simulink library "speedgoatlib_mscp"  (R2024b)
settings: Solver=VariableStepAuto  StartTime=0.0  StopTime=10.0  RelTol=1e-3
libraries: slrealtimeethercatlib x517, simulink x316, hdlsllib x168, $bdroot x11, slrealtimeutilitieslib x1
(part 1 of 5)
settings Model: Creator=lars.brockmann  LastModifiedBy=speedgoat\jenkins
settings ConfigComp: CovBoundaryAbsTol=1.0e-5

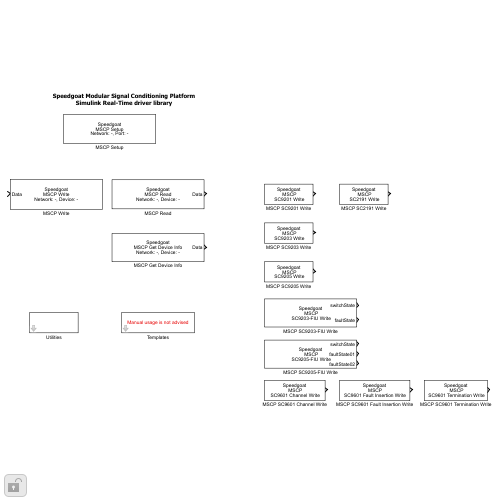
[thumbnail: Simulink's stored preview of the top-level diagram]
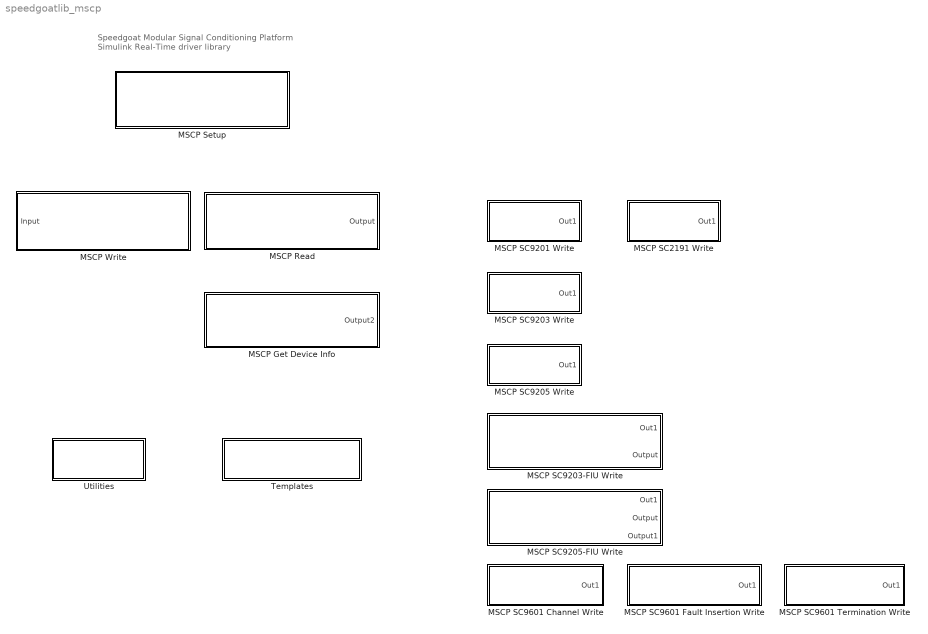
== system speedgoatlib_mscp ==
  note: Speedgoat Modular Signal Conditioning Platform
      | Simulink Real-Time driver library
  MSCP Get Device Info : Subsystem  mask(mscp_getDeviceInfo){}
      settings: OpenFcn=sg_mscp.mask.openFcn('MSCP Get Device Info');
      mask Help: eval('sg.utils.help.show(''io_main/refentry_mscp_get_device_info'');')
      mask Display: disp('Speedgoat\nMSCP Get Device Info\nNetwork: -, Device: -');port_label('output',1,'Data');
  MSCP Read : Subsystem  mask(mscp_read){}
      settings: OpenFcn=sg_mscp.mask.openFcn('MSCP Read');
      mask Help: eval('sg.utils.help.show(''io_main/refentry_mscp_read'');')
      mask Display: disp('Speedgoat\nMSCP Read\nNetwork: -, Device: -');port_label('output',1,'Data');
  MSCP SC2191 Write : Subsystem  mask(mscp_sc2191_write){}
      settings: OpenFcn=sg_mscp.mask.openFcn('MSCP SC2191 Write')
      mask Help: eval('sg.utils.help.show(''io_main/refentry_mscp_sc2191'');')
      mask Display: disp('Speedgoat\n MSCP\n SC2191 Write')
  MSCP SC9201 Write : Subsystem  mask(mscp_sc9201_write){switchState=0}
      settings: OpenFcn=sg_mscp.mask.openFcn(['MSCP SC9201 Write (',gcb,')'])
      mask Help: eval('sg.utils.help.show(''io_main/refentry_mscp_sc9201'');')
      mask Display: disp('Speedgoat\n MSCP\n SC9201 Write')
  MSCP SC9203 Write : Subsystem  mask(mscp_sc9203_write){switchState=0}
      settings: OpenFcn=sg_mscp.mask.openFcn(['MSCP SC9203 Write (',gcb,')'])
      mask Help: eval('sg.utils.help.show(''io_main/refentry_mscp_sc9203'');')
      mask Display: disp('Speedgoat\n MSCP\n SC9203 Write')
  MSCP SC9203-FIU Write : Subsystem  mask(mscp_sc9203_fiu_write){switchState=0, faultState=0}
      settings: OpenFcn=sg_mscp.mask.openFcn(['MSCP SC9203-FIU Write (',gcb,')'])
      mask Help: eval('sg.utils.help.show(''io_main/refentry_mscp_sc9203_fiu'');')
      mask Display:
      | port_label('output', 1, 'switchState');
      | port_label('output', 2, 'faultState');
      | disp('Speedgoat\n MSCP\n SC9203-FIU Write')
  MSCP SC9205 Write : Subsystem  mask(mscp_sc9205_write){switchState=0}
      settings: OpenFcn=sg_mscp.mask.openFcn(['MSCP SC9205 Write (',gcb,')'])
      mask Help: eval('sg.utils.help.show(''io_main/refentry_mscp_sc9205'');')
      mask Display: disp('Speedgoat\n MSCP\n SC9205 Write')
  MSCP SC9205-FIU Write : Subsystem  mask(mscp_sc9205_fiu_write){switchState=0, faultState01=0, faultState02=0}
      settings: OpenFcn=sg_mscp.mask.openFcn(['MSCP SC9205-FIU Write (',gcb,')'])
      mask Help: eval('sg.utils.help.show(''io_main/refentry_mscp_sc9205_fiu'');')
      mask Display:
      | port_label('output', 1, 'switchState');
      | port_label('output', 2, 'faultState01');
      | port_label('output', 3, 'faultState02');
      | disp('Speedgoat\n MSCP\n SC9205-FIU Write')
  MSCP SC9601 Channel Write : Subsystem  mask(mscp_sc9601_channel_write){switchState=0}
      settings: OpenFcn=sg_mscp.mask.openFcn;
      mask Help: eval('sg.utils.help.show(''io_main/refentry_ref_mscp'');')
      mask Display: disp('Speedgoat\n MSCP\n SC9601 Channel Write')
  MSCP SC9601 Fault Insertion Write : Subsystem  mask(mscp_sc9601_fault_insertion_write){switchState=0}
      settings: OpenFcn=sg_mscp.mask.openFcn;
      mask Help: eval('sg.utils.help.show(''io_main/refentry_ref_mscp'');')
      mask Display: disp('Speedgoat\n MSCP\n SC9601 Fault Insertion Write')
  MSCP SC9601 Termination Write : Subsystem  mask(mscp_sc9601_termination_write){switchState=0}
      settings: OpenFcn=sg_mscp.mask.openFcn;
      mask Help: eval('sg.utils.help.show(''io_main/refentry_ref_mscp'');')
      mask Display: disp('Speedgoat\n MSCP\n SC9601 Termination Write')
  MSCP Setup : Subsystem  mask(mscp_setup){}
      settings: OpenFcn=sg_mscp.mask.openFcn('MSCP Setup');
      mask Help: eval('sg.utils.help.show(''io_main/refentry_mscp_setup'');')
      mask Display: disp('Speedgoat\nMSCP Setup\nNetwork: -, Port: -');
  MSCP Write : Subsystem  mask(mscp_write){}
      settings: OpenFcn=sg_mscp.mask.openFcn('MSCP Write');
      mask Help: eval('sg.utils.help.show(''io_main/refentry_mscp_write'');')
      mask Display: disp('Speedgoat\nMSCP Write\nNetwork: -, Device: -');port_label('input',1,'Data');
  Templates : Subsystem
      mask Display:
      | color('red');
      | disp('Manual usage is not advised');
  Utilities : Subsystem

== system speedgoatlib_mscp/MSCP Get Device Info ==
  Bus Creator : BusCreator  Inputs=12
  Subsystem Device : Subsystem  Commented=on
  Subsystem Slot 01 : Subsystem  Commented=on
  Subsystem Slot 02 : Subsystem  Commented=on
  Subsystem Slot 03 : Subsystem  Commented=on
  Subsystem Slot 04 : Subsystem  Commented=on
  Subsystem Slot 05 : Subsystem  Commented=on
  Subsystem Slot 06 : Subsystem  Commented=on
  Subsystem Slot 07 : Subsystem  Commented=on
  Subsystem Slot 08 : Subsystem  Commented=on
  Subsystem Slot 09 : Subsystem  Commented=on
  Subsystem Slot 10 : Subsystem  Commented=on
  Subsystem Slot 11 : Subsystem  Commented=on
  Output2 : Outport
  wires:
  Subsystem Slot 01/1(Out1) -> Bus Creator/2  "Slot_01"
  Subsystem Slot 02/1(Out1) -> Bus Creator/3  "Slot_02"
  Subsystem Slot 03/1(Out1) -> Bus Creator/4  "Slot_03"
  Subsystem Slot 04/1(Out1) -> Bus Creator/5  "Slot_04"
  Subsystem Slot 05/1(Out1) -> Bus Creator/6  "Slot_05"
  Subsystem Slot 06/1(Out1) -> Bus Creator/7  "Slot_06"
  Subsystem Slot 07/1(Out1) -> Bus Creator/8  "Slot_07"
  Subsystem Slot 08/1(Out1) -> Bus Creator/9  "Slot_08"
  Subsystem Slot 09/1(Out1) -> Bus Creator/10  "Slot_09"
  Subsystem Slot 10/1(Out1) -> Bus Creator/11  "Slot_10"
  Subsystem Slot 11/1(Out1) -> Bus Creator/12  "Slot_11"
  Bus Creator/1 -> Output2/1  "Data"
  Subsystem Device/1(Out1) -> Bus Creator/1  "Device"

== system speedgoatlib_mscp/MSCP Read ==
  Output : Outport

== system speedgoatlib_mscp/MSCP SC2191 Write ==
  Configuration : Constant  Value=0  OutDataTypeStr=Bus: MscpBus_SC2191_Write
  Out1 : Outport
  wires:
  Configuration/1 -> Out1/1

== system speedgoatlib_mscp/MSCP SC9201 Write ==
  Constant : Constant  Value=switchState  OutDataTypeStr=uint8
  Out1 : Outport
  wires:
  Constant/1 -> Out1/1

== system speedgoatlib_mscp/MSCP SC9203 Write ==
  Constant : Constant  Value=switchState  OutDataTypeStr=uint8
  Out1 : Outport
  wires:
  Constant/1 -> Out1/1

== system speedgoatlib_mscp/MSCP SC9203-FIU Write ==
  Constant : Constant  Value=switchState  OutDataTypeStr=uint8
  Constant1 : Constant  Value=faultState  OutDataTypeStr=uint8
  Out1 : Outport
  Output : Outport  Port=2
  wires:
  Constant/1 -> Out1/1
  Constant1/1 -> Output/1

== system speedgoatlib_mscp/MSCP SC9205 Write ==
  Constant : Constant  Value=switchState  OutDataTypeStr=uint8
  Out1 : Outport
  wires:
  Constant/1 -> Out1/1

== system speedgoatlib_mscp/MSCP SC9205-FIU Write ==
  Constant : Constant  Value=switchState  OutDataTypeStr=uint8
  Constant1 : Constant  Value=faultState01  OutDataTypeStr=uint8
  Constant2 : Constant  Value=faultState02  OutDataTypeStr=uint8
  Out1 : Outport
  Output : Outport  Port=2
  Output1 : Outport  Port=3
  wires:
  Constant1/1 -> Output/1
  Constant/1 -> Out1/1
  Constant2/1 -> Output1/1

== system speedgoatlib_mscp/MSCP SC9601 Channel Write ==
  Constant : Constant  Value=switchState  OutDataTypeStr=uint8
  Out1 : Outport
  wires:
  Constant/1 -> Out1/1

== system speedgoatlib_mscp/MSCP SC9601 Fault Insertion Write ==
  Constant : Constant  Value=switchState  OutDataTypeStr=uint8
  Out1 : Outport
  wires:
  Constant/1 -> Out1/1

== system speedgoatlib_mscp/MSCP SC9601 Termination Write ==
  Constant : Constant  Value=switchState  OutDataTypeStr=uint8
  Out1 : Outport
  wires:
  Constant/1 -> Out1/1

== system speedgoatlib_mscp/MSCP Setup ==
  Constant : Constant
  Terminator : Terminator
  wires:
  Constant/1 -> Terminator/1

== system speedgoatlib_mscp/MSCP Write ==
  Input : Inport
  Terminator : Terminator
  wires:
  Input/1 -> Terminator/1

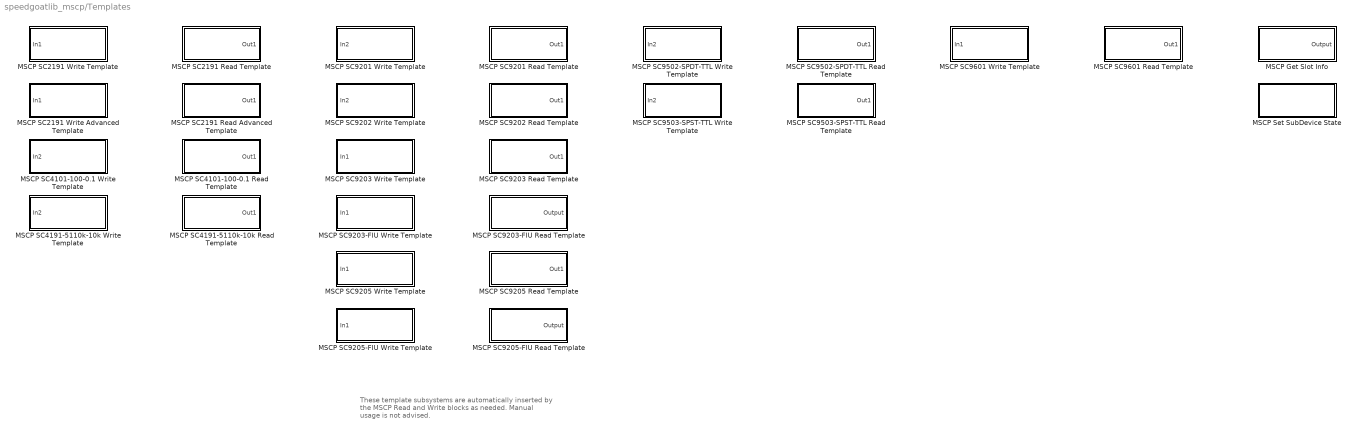
== system speedgoatlib_mscp/Templates ==
  note: These template subsystems are automatically inserted
      | by the MSCP Read and Write blocks as needed.
      | Manual usage is not advised.
  MSCP Get Slot Info : Subsystem
  MSCP SC2191 Read Advanced Template : Subsystem
  MSCP SC2191 Read Template : Subsystem
  MSCP SC2191 Write Advanced Template : Subsystem
  MSCP SC2191 Write Template : Subsystem
  MSCP SC4101-100-0.1 Read Template : Subsystem
  MSCP SC4101-100-0.1 Write Template : Subsystem
  MSCP SC4191-5110k-10k Read Template : Subsystem
  MSCP SC4191-5110k-10k Write Template : Subsystem
  MSCP SC9201 Read Template : Subsystem
  MSCP SC9201 Write Template : Subsystem
  MSCP SC9202 Read Template : Subsystem
  MSCP SC9202 Write Template : Subsystem
  MSCP SC9203 Read Template : Subsystem
  MSCP SC9203 Write Template : Subsystem
  MSCP SC9203-FIU Read Template : Subsystem
  MSCP SC9203-FIU Write Template : Subsystem
  MSCP SC9205 Read Template : Subsystem
  MSCP SC9205 Write Template : Subsystem
  MSCP SC9205-FIU Read Template : Subsystem
  MSCP SC9205-FIU Write Template : Subsystem
  MSCP SC9502-SPDT-TTL Read Template : Subsystem
  MSCP SC9502-SPDT-TTL Write Template : Subsystem
  MSCP SC9503-SPST-TTL Read Template : Subsystem
  MSCP SC9503-SPST-TTL Write Template : Subsystem
  MSCP SC9601 Read Template : Subsystem
  MSCP SC9601 Write Template : Subsystem
  MSCP Set SubDevice State : Subsystem

== system speedgoatlib_mscp/Utilities ==
  MSCP Parse Emergency : S-Function  FunctionName=sg_mscp_parse_ecat_emergency  SFunctionDeploymentMode=off  EnableBusSupport=off
  MSCP Parse Notifications : S-Function  FunctionName=sg_mscp_parse_ecat_notifications  SFunctionDeploymentMode=off  EnableBusSupport=off

== system speedgoatlib_mscp/MSCP Get Device Info/Subsystem Device ==
  ASCII to String : ASCIIToString
  ASCII to String1 : ASCIIToString
  Bus Creator : BusCreator  Inputs=2
  Cast : DataTypeConversion  OutDataTypeStr=int32  SaturateOnIntegerOverflow=off  RndMeth=Floor
  Compare To Constant : simulink/Logic and Bit Operations/Compare To Constant  relop=>=  const=2  OutDataTypeStr=boolean
  EtherCAT Async SDO Upload 0x1008 : slrealtimeethercatlib/EtherCAT Async SDO Upload  index=0  subIndex=0  sig_type=uint8  sig_dim=16  device_id=0  sample_time=1  subdevice_addr=0  selected_subdevice=Term 1 (EK1100)  timeout=500  subdevice_found=0  complete=0
  EtherCAT Async SDO Upload 0x100A : slrealtimeethercatlib/EtherCAT Async SDO Upload  index=0  subIndex=0  sig_type=uint8  sig_dim=16  device_id=0  sample_time=1  subdevice_addr=0  selected_subdevice=Term 1 (EK1100)  timeout=500  subdevice_found=0  complete=0
  Get SubDevice State : slrealtimeethercatlib/Get SubDevice State  device_id=0  sample_time=1  subdevice_addr=0  selected_subdevice=Term 1 (EK1100)  timeout=500  subdevice_found=0
  Terminator{2..5} (4 alike) : Terminator
  Out1 : Outport
  wires:
  Bus Creator/1 -> Out1/1
  EtherCAT Async SDO Upload 0x100A/3 -> Terminator2/1
  EtherCAT Async SDO Upload 0x100A/2 -> Terminator3/1
  EtherCAT Async SDO Upload 0x1008/3 -> Terminator4/1
  EtherCAT Async SDO Upload 0x1008/2 -> Terminator5/1
  Get SubDevice State/1 -> Compare To Constant/1
  Compare To Constant/1 -> Cast/1
  Cast/1 -> EtherCAT Async SDO Upload 0x1008/1, EtherCAT Async SDO Upload 0x100A/1
  ASCII to String/1 -> Bus Creator/2  "Software Version"
  EtherCAT Async SDO Upload 0x100A/1 -> ASCII to String/1
  ASCII to String1/1 -> Bus Creator/1  "Manufacturer Device Name"
  EtherCAT Async SDO Upload 0x1008/1 -> ASCII to String1/1

== system speedgoatlib_mscp/MSCP Get Device Info/Subsystem Slot 01 ==
  MSCP Get Slot Info : $bdroot/Templates/MSCP Get Slot Info  SystemSampleTime=-1  VariantActivationTime=update diagram  EmptyChoice=off  PassThrough=off  PassThroughVariantControl=(default)  EmptyChoiceVariantControl=(default)  AllowFlexibleInterface=on  Latency=0  AutoFrameSizeCalculation=off
  Out1 : Outport
  wires:
  MSCP Get Slot Info/1 -> Out1/1

== system speedgoatlib_mscp/MSCP Get Device Info/Subsystem Slot 02 ==
  MSCP Get Slot Info : $bdroot/Templates/MSCP Get Slot Info  SystemSampleTime=-1  VariantActivationTime=update diagram  EmptyChoice=off  PassThrough=off  PassThroughVariantControl=(default)  EmptyChoiceVariantControl=(default)  AllowFlexibleInterface=on  Latency=0  AutoFrameSizeCalculation=off
  Out1 : Outport
  wires:
  MSCP Get Slot Info/1 -> Out1/1

== system speedgoatlib_mscp/MSCP Get Device Info/Subsystem Slot 03 ==
  MSCP Get Slot Info : $bdroot/Templates/MSCP Get Slot Info  SystemSampleTime=-1  VariantActivationTime=update diagram  EmptyChoice=off  PassThrough=off  PassThroughVariantControl=(default)  EmptyChoiceVariantControl=(default)  AllowFlexibleInterface=on  Latency=0  AutoFrameSizeCalculation=off
  Out1 : Outport
  wires:
  MSCP Get Slot Info/1 -> Out1/1

== system speedgoatlib_mscp/MSCP Get Device Info/Subsystem Slot 04 ==
  MSCP Get Slot Info : $bdroot/Templates/MSCP Get Slot Info  SystemSampleTime=-1  VariantActivationTime=update diagram  EmptyChoice=off  PassThrough=off  PassThroughVariantControl=(default)  EmptyChoiceVariantControl=(default)  AllowFlexibleInterface=on  Latency=0  AutoFrameSizeCalculation=off
  Out1 : Outport
  wires:
  MSCP Get Slot Info/1 -> Out1/1

== system speedgoatlib_mscp/MSCP Get Device Info/Subsystem Slot 05 ==
  MSCP Get Slot Info : $bdroot/Templates/MSCP Get Slot Info  SystemSampleTime=-1  VariantActivationTime=update diagram  EmptyChoice=off  PassThrough=off  PassThroughVariantControl=(default)  EmptyChoiceVariantControl=(default)  AllowFlexibleInterface=on  Latency=0  AutoFrameSizeCalculation=off
  Out1 : Outport
  wires:
  MSCP Get Slot Info/1 -> Out1/1

== system speedgoatlib_mscp/MSCP Get Device Info/Subsystem Slot 06 ==
  MSCP Get Slot Info : $bdroot/Templates/MSCP Get Slot Info  SystemSampleTime=-1  VariantActivationTime=update diagram  EmptyChoice=off  PassThrough=off  PassThroughVariantControl=(default)  EmptyChoiceVariantControl=(default)  AllowFlexibleInterface=on  Latency=0  AutoFrameSizeCalculation=off
  Out1 : Outport
  wires:
  MSCP Get Slot Info/1 -> Out1/1

== system speedgoatlib_mscp/MSCP Get Device Info/Subsystem Slot 07 ==
  MSCP Get Slot Info : $bdroot/Templates/MSCP Get Slot Info  SystemSampleTime=-1  VariantActivationTime=update diagram  EmptyChoice=off  PassThrough=off  PassThroughVariantControl=(default)  EmptyChoiceVariantControl=(default)  AllowFlexibleInterface=on  Latency=0  AutoFrameSizeCalculation=off
  Out1 : Outport
  wires:
  MSCP Get Slot Info/1 -> Out1/1

== system speedgoatlib_mscp/MSCP Get Device Info/Subsystem Slot 08 ==
  MSCP Get Slot Info : $bdroot/Templates/MSCP Get Slot Info  SystemSampleTime=-1  VariantActivationTime=update diagram  EmptyChoice=off  PassThrough=off  PassThroughVariantControl=(default)  EmptyChoiceVariantControl=(default)  AllowFlexibleInterface=on  Latency=0  AutoFrameSizeCalculation=off
  Out1 : Outport
  wires:
  MSCP Get Slot Info/1 -> Out1/1

== system speedgoatlib_mscp/MSCP Get Device Info/Subsystem Slot 09 ==
  MSCP Get Slot Info : $bdroot/Templates/MSCP Get Slot Info  SystemSampleTime=-1  VariantActivationTime=update diagram  EmptyChoice=off  PassThrough=off  PassThroughVariantControl=(default)  EmptyChoiceVariantControl=(default)  AllowFlexibleInterface=on  Latency=0  AutoFrameSizeCalculation=off
  Out1 : Outport
  wires:
  MSCP Get Slot Info/1 -> Out1/1

== system speedgoatlib_mscp/MSCP Get Device Info/Subsystem Slot 10 ==
  MSCP Get Slot Info : $bdroot/Templates/MSCP Get Slot Info  SystemSampleTime=-1  VariantActivationTime=update diagram  EmptyChoice=off  PassThrough=off  PassThroughVariantControl=(default)  EmptyChoiceVariantControl=(default)  AllowFlexibleInterface=on  Latency=0  AutoFrameSizeCalculation=off
  Out1 : Outport
  wires:
  MSCP Get Slot Info/1 -> Out1/1

== system speedgoatlib_mscp/MSCP Get Device Info/Subsystem Slot 11 ==
  MSCP Get Slot Info : $bdroot/Templates/MSCP Get Slot Info  SystemSampleTime=-1  VariantActivationTime=update diagram  EmptyChoice=off  PassThrough=off  PassThroughVariantControl=(default)  EmptyChoiceVariantControl=(default)  AllowFlexibleInterface=on  Latency=0  AutoFrameSizeCalculation=off
  Out1 : Outport
  wires:
  MSCP Get Slot Info/1 -> Out1/1

== system speedgoatlib_mscp/Templates/MSCP Get Slot Info ==
  ASCII to String{,1..3} (4 alike) : ASCIIToString
  Bus Creator : BusCreator  Inputs=9
  Byte Unpacking : slrealtimeutilitieslib/Byte Unpacking  MaskUnpackedDataTypes={'uint16', 'boolean', 'uint8', 'uint8', 'uint8', 'uint32','uint8', 'int64', 'uint8', 'uint16'}  MaskUnpackedDataSizes={[1], [1], [1], [32], [64], [1], [16], [1], [32],[1]}  MaskAlignment=1
  Cast : DataTypeConversion  OutDataTypeStr=int32  SaturateOnIntegerOverflow=off  RndMeth=Floor
  Compare To Constant : simulink/Logic and Bit Operations/Compare To Constant  relop=>=  const=2  OutDataTypeStr=boolean
  EtherCAT Async SDO Upload : slrealtimeethercatlib/EtherCAT Async SDO Upload  index=0  subIndex=0  sig_type=uint8  sig_dim=162  device_id=0  sample_time=1  subdevice_addr=0  selected_subdevice=Term 1 (EK1100)  timeout=500  subdevice_found=0  complete=0
  Get SubDevice State : slrealtimeethercatlib/Get SubDevice State  device_id=0  sample_time=1  subdevice_addr=0  selected_subdevice=Term 1 (EK1100)  timeout=500  subdevice_found=0
  Terminator : Terminator
  Terminator1 : Terminator
  Terminator2 : Terminator
  To String : ToString
  Output : Outport
  wires:
  Cast/1 -> EtherCAT Async SDO Upload/1
  Get SubDevice State/1 -> Compare To Constant/1
  Compare To Constant/1 -> Cast/1
  EtherCAT Async SDO Upload/2 -> Terminator1/1
  Byte Unpacking/3 -> Bus Creator/2  "Header Layout Version"
  Byte Unpacking/1 -> Terminator/1  "number of subobjects"
  EtherCAT Async SDO Upload/3 -> Terminator2/1
  Byte Unpacking/6 -> Bus Creator/5  "Module Identificaiton Number"
  Byte Unpacking/2 -> Bus Creator/1  "Header Control Byte"
  EtherCAT Async SDO Upload/1 -> Byte Unpacking/1
  ASCII to String/1 -> Bus Creator/4  "Notes"
  Byte Unpacking/5 -> ASCII to String/1
  Bus Creator/1 -> Output/1
  Byte Unpacking/7 -> ASCII to String1/1
  ASCII to String1/1 -> Bus Creator/6  "Hardware Version"
  Byte Unpacking/4 -> ASCII to String2/1
  ASCII to String2/1 -> Bus Creator/3  "Product Name"
  Byte Unpacking/8 -> To String/1
  To String/1 -> Bus Creator/7  "Flash Date"
  Byte Unpacking/9 -> ASCII to String3/1
  ASCII to String3/1 -> Bus Creator/8  "Serial Number"
  Byte Unpacking/10 -> Bus Creator/9  "CRC Residue"

== system speedgoatlib_mscp/Templates/MSCP SC2191 Read Advanced Template ==
  Bus Creator : BusCreator  Inputs=16  OutDataTypeStr=Bus: MscpBus_SC2191_Advanced_Read
      settings: InheritFromInputs=off
  Channel_01 : Subsystem
  Channel_02 : Subsystem
  Channel_03 : Subsystem
  Channel_04 : Subsystem
  Channel_05 : Subsystem
  Channel_06 : Subsystem
  Channel_07 : Subsystem
  Channel_08 : Subsystem
  Channel_09 : Subsystem
  Channel_10 : Subsystem
  Channel_11 : Subsystem
  Channel_12 : Subsystem
  Channel_13 : Subsystem
  Channel_14 : Subsystem
  Channel_15 : Subsystem
  Channel_16 : Subsystem
  Out1 : Outport
  wires:
  Channel_16/1(Out1) -> Bus Creator/16  "Channel_16"
  Channel_15/1(Out1) -> Bus Creator/15  "Channel_15"
  Channel_14/1(Out1) -> Bus Creator/14  "Channel_14"
  Channel_13/1(Out1) -> Bus Creator/13  "Channel_13"
  Channel_12/1(Out1) -> Bus Creator/12  "Channel_12"
  Channel_11/1(Out1) -> Bus Creator/11  "Channel_11"
  Channel_10/1(Out1) -> Bus Creator/10  "Channel_10"
  Channel_09/1(Out1) -> Bus Creator/9  "Channel_09"
  Channel_08/1(Out1) -> Bus Creator/8  "Channel_08"
  Channel_07/1(Out1) -> Bus Creator/7  "Channel_07"
  Channel_06/1(Out1) -> Bus Creator/6  "Channel_06"
  Channel_05/1(Out1) -> Bus Creator/5  "Channel_05"
  Channel_04/1(Out1) -> Bus Creator/4  "Channel_04"
  Channel_03/1(Out1) -> Bus Creator/3  "Channel_03"
  Channel_02/1(Out1) -> Bus Creator/2  "Channel_02"
  Channel_01/1(Out1) -> Bus Creator/1  "Channel_01"
  Bus Creator/1 -> Out1/1

== system speedgoatlib_mscp/Templates/MSCP SC2191 Read Template ==
  Bus Creator : BusCreator  Inputs=16  OutDataTypeStr=Bus: MscpBus_SC2191_Read
      settings: InheritFromInputs=off
  Channel_01 : Subsystem
  Channel_02 : Subsystem
  Channel_03 : Subsystem
  Channel_04 : Subsystem
  Channel_05 : Subsystem
  Channel_06 : Subsystem
  Channel_07 : Subsystem
  Channel_08 : Subsystem
  Channel_09 : Subsystem
  Channel_10 : Subsystem
  Channel_11 : Subsystem
  Channel_12 : Subsystem
  Channel_13 : Subsystem
  Channel_14 : Subsystem
  Channel_15 : Subsystem
  Channel_16 : Subsystem
  Out1 : Outport
  wires:
  Bus Creator/1 -> Out1/1
  Channel_01/1(Out1) -> Bus Creator/1  "Channel_01"
  Channel_02/1(Out1) -> Bus Creator/2  "Channel_02"
  Channel_03/1(Out1) -> Bus Creator/3  "Channel_03"
  Channel_04/1(Out1) -> Bus Creator/4  "Channel_04"
  Channel_05/1(Out1) -> Bus Creator/5  "Channel_05"
  Channel_06/1(Out1) -> Bus Creator/6  "Channel_06"
  Channel_07/1(Out1) -> Bus Creator/7  "Channel_07"
  Channel_08/1(Out1) -> Bus Creator/8  "Channel_08"
  Channel_09/1(Out1) -> Bus Creator/9  "Channel_09"
  Channel_10/1(Out1) -> Bus Creator/10  "Channel_10"
  Channel_11/1(Out1) -> Bus Creator/11  "Channel_11"
  Channel_12/1(Out1) -> Bus Creator/12  "Channel_12"
  Channel_13/1(Out1) -> Bus Creator/13  "Channel_13"
  Channel_14/1(Out1) -> Bus Creator/14  "Channel_14"
  Channel_15/1(Out1) -> Bus Creator/15  "Channel_15"
  Channel_16/1(Out1) -> Bus Creator/16  "Channel_16"

== system speedgoatlib_mscp/Templates/MSCP SC2191 Write Advanced Template ==
  In1 : Inport  OutDataTypeStr=Bus: MscpBus_SC2191_Advanced_Write
  Bus Selector : BusSelector  OutputSignals=Channel_01,Channel_02,Channel_03,Channel_04,Channel_05,Channel_06,Channel_07,Channel_08,Channel_09,Channel_10,Channel_11,Channel_12,Channel_13,Channel_14,Channel_15,Channel_16
  Channel_01 : Subsystem
  Channel_02 : Subsystem
  Channel_03 : Subsystem
  Channel_04 : Subsystem
  Channel_05 : Subsystem
  Channel_06 : Subsystem
  Channel_07 : Subsystem
  Channel_08 : Subsystem
  Channel_09 : Subsystem
  Channel_10 : Subsystem
  Channel_11 : Subsystem
  Channel_12 : Subsystem
  Channel_13 : Subsystem
  Channel_14 : Subsystem
  Channel_15 : Subsystem
  Channel_16 : Subsystem
  wires:
  Bus Selector/16 -> Channel_16/1(In1)  "<Channel_16>"
  Bus Selector/15 -> Channel_15/1(In1)  "<Channel_15>"
  Bus Selector/14 -> Channel_14/1(In1)  "<Channel_14>"
  Bus Selector/13 -> Channel_13/1(In1)  "<Channel_13>"
  Bus Selector/12 -> Channel_12/1(In1)  "<Channel_12>"
  Bus Selector/11 -> Channel_11/1(In1)  "<Channel_11>"
  Bus Selector/10 -> Channel_10/1(In1)  "<Channel_10>"
  Bus Selector/9 -> Channel_09/1(In1)  "<Channel_09>"
  Bus Selector/8 -> Channel_08/1(In1)  "<Channel_08>"
  Bus Selector/7 -> Channel_07/1(In1)  "<Channel_07>"
  Bus Selector/6 -> Channel_06/1(In1)  "<Channel_06>"
  Bus Selector/5 -> Channel_05/1(In1)  "<Channel_05>"
  Bus Selector/4 -> Channel_04/1(In1)  "<Channel_04>"
  Bus Selector/3 -> Channel_03/1(In1)  "<Channel_03>"
  Bus Selector/2 -> Channel_02/1(In1)  "<Channel_02>"
  Bus Selector/1 -> Channel_01/1(In1)  "<Channel_01>"
  In1/1 -> Bus Selector/1

== system speedgoatlib_mscp/Templates/MSCP SC2191 Write Template ==
  In1 : Inport  OutDataTypeStr=Bus: MscpBus_SC2191_Write
  Bus Selector : BusSelector  OutputSignals=Channel_01,Channel_02,Channel_03,Channel_04,Channel_05,Channel_06,Channel_07,Channel_08,Channel_09,Channel_10,Channel_11,Channel_12,Channel_13,Channel_14,Channel_15,Channel_16
  Channel_01 : Subsystem
  Channel_02 : Subsystem
  Channel_03 : Subsystem
  Channel_04 : Subsystem
  Channel_05 : Subsystem
  Channel_06 : Subsystem
  Channel_07 : Subsystem
  Channel_08 : Subsystem
  Channel_09 : Subsystem
  Channel_10 : Subsystem
  Channel_11 : Subsystem
  Channel_12 : Subsystem
  Channel_13 : Subsystem
  Channel_14 : Subsystem
  Channel_15 : Subsystem
  Channel_16 : Subsystem
  wires:
  In1/1 -> Bus Selector/1
  Bus Selector/1 -> Channel_01/1(In1)  "<Channel_01>"
  Bus Selector/2 -> Channel_02/1(In1)  "<Channel_02>"
  Bus Selector/3 -> Channel_03/1(In1)  "<Channel_03>"
  Bus Selector/4 -> Channel_04/1(In1)  "<Channel_04>"
  Bus Selector/5 -> Channel_05/1(In1)  "<Channel_05>"
  Bus Selector/6 -> Channel_06/1(In1)  "<Channel_06>"
  Bus Selector/7 -> Channel_07/1(In1)  "<Channel_07>"
  Bus Selector/8 -> Channel_08/1(In1)  "<Channel_08>"
  Bus Selector/9 -> Channel_09/1(In1)  "<Channel_09>"
  Bus Selector/10 -> Channel_10/1(In1)  "<Channel_10>"
  Bus Selector/11 -> Channel_11/1(In1)  "<Channel_11>"
  Bus Selector/12 -> Channel_12/1(In1)  "<Channel_12>"
  Bus Selector/13 -> Channel_13/1(In1)  "<Channel_13>"
  Bus Selector/14 -> Channel_14/1(In1)  "<Channel_14>"
  Bus Selector/15 -> Channel_15/1(In1)  "<Channel_15>"
  Bus Selector/16 -> Channel_16/1(In1)  "<Channel_16>"

== system speedgoatlib_mscp/Templates/MSCP SC4101-100-0.1 Read Template ==
  Bus Creator : BusCreator  Inputs=8  OutDataTypeStr=Bus: MscpBus_SC4101_100_0_1
      settings: InheritFromInputs=off
  S-Function : S-Function  FunctionName=sg_mscp_SC4101_100_0_1_read  SFunctionDeploymentMode=off  EnableBusSupport=off
  exp0bank{0..4} (5 alike) : slrealtimeethercatlib/EtherCAT PDO Receive  Priority=2  sig_name=Uninitialized Block  sig_offset=144  sig_type=uint8  type_size=8  sig_dim=1  device_id=0  sample_time=0.010000
  exp1bank{0..4} (5 alike) : slrealtimeethercatlib/EtherCAT PDO Receive  Priority=2  sig_name=Uninitialized Block  sig_offset=144  sig_type=uint8  type_size=8  sig_dim=1  device_id=0  sample_time=0.010000
  Out1 : Outport
  wires:
  exp0bank3/1 -> S-Function/4
  exp1bank0/1 -> S-Function/6
  Bus Creator/1 -> Out1/1
  exp0bank2/1 -> S-Function/3
  exp0bank0/1 -> S-Function/1
  exp1bank1/1 -> S-Function/7
  exp0bank1/1 -> S-Function/2
  exp0bank4/1 -> S-Function/5
  S-Function/1 -> Bus Creator/1  "Channel_01"
  S-Function/2 -> Bus Creator/2  "Channel_02"
  S-Function/3 -> Bus Creator/3  "Channel_03"
  S-Function/4 -> Bus Creator/4  "Channel_04"
  S-Function/5 -> Bus Creator/5  "Channel_05"
  S-Function/6 -> Bus Creator/6  "Channel_06"
  S-Function/7 -> Bus Creator/7  "Channel_07"
  S-Function/8 -> Bus Creator/8  "Channel_08"
  exp1bank2/1 -> S-Function/8
  exp1bank3/1 -> S-Function/9
  exp1bank4/1 -> S-Function/10

== system speedgoatlib_mscp/Templates/MSCP SC4101-100-0.1 Write Template ==
  In2 : Inport  OutDataTypeStr=Bus: MscpBus_SC4101_100_0_1
  Bus Selector1 : BusSelector  OutputSignals=Channel_01,Channel_02,Channel_03,Channel_04,Channel_05,Channel_06,Channel_07,Channel_08
  S-Function : S-Function  FunctionName=sg_mscp_SC4101_100_0_1_write  SFunctionDeploymentMode=off  EnableBusSupport=off
  exp0bank{0..4} (5 alike) : slrealtimeethercatlib/EtherCAT PDO Transmit  Priority=3  sig_name=Uninitialized Block  sig_offset=128  sig_type=uint8  type_size=8  sig_dim=1  device_id=0  sample_time=0.010000
  exp1bank{0..4} (5 alike) : slrealtimeethercatlib/EtherCAT PDO Transmit  Priority=3  sig_name=Uninitialized Block  sig_offset=128  sig_type=uint8  type_size=8  sig_dim=1  device_id=0  sample_time=0.010000
  wires:
  Bus Selector1/4 -> S-Function/4  "<Channel_04>"
  Bus Selector1/3 -> S-Function/3  "<Channel_03>"
  Bus Selector1/5 -> S-Function/5  "<Channel_05>"
  In2/1 -> Bus Selector1/1
  Bus Selector1/2 -> S-Function/2  "<Channel_02>"
  Bus Selector1/6 -> S-Function/6  "<Channel_06>"
  Bus Selector1/7 -> S-Function/7  "<Channel_07>"
  Bus Selector1/1 -> S-Function/1  "<Channel_01>"
  Bus Selector1/8 -> S-Function/8  "<Channel_08>"
  S-Function/1 -> exp0bank0/1
  S-Function/2 -> exp0bank1/1
  S-Function/3 -> exp0bank2/1
  S-Function/4 -> exp0bank3/1
  S-Function/5 -> exp0bank4/1
  S-Function/6 -> exp1bank0/1
  S-Function/7 -> exp1bank1/1
  S-Function/8 -> exp1bank2/1
  S-Function/9 -> exp1bank3/1
  S-Function/10 -> exp1bank4/1

== system speedgoatlib_mscp/Templates/MSCP SC4191-5110k-10k Read Template ==
  Bus Creator : BusCreator  Inputs=1  OutDataTypeStr=Bus: MscpBus_SC4191_5110k_10k
      settings: InheritFromInputs=off
  S-Function1 : S-Function  FunctionName=sg_mscp_SC4191_5110k_10k_read  SFunctionDeploymentMode=off  EnableBusSupport=off
  exp0bank0 : slrealtimeethercatlib/EtherCAT PDO Receive  Priority=2  sig_name=Uninitialized Block  sig_offset=144  sig_type=uint8  type_size=8  sig_dim=1  device_id=0  sample_time=0.010000
  exp0bank1 : slrealtimeethercatlib/EtherCAT PDO Receive  Priority=2  sig_name=Uninitialized Block  sig_offset=144  sig_type=uint8  type_size=8  sig_dim=1  device_id=0  sample_time=0.010000
  Out1 : Outport
  wires:
  exp0bank0/1 -> S-Function1/1
  exp0bank1/1 -> S-Function1/2
  Bus Creator/1 -> Out1/1
  S-Function1/1 -> Bus Creator/1  "Channel_01"

== system speedgoatlib_mscp/Templates/MSCP SC4191-5110k-10k Write Template ==
  In2 : Inport  OutDataTypeStr=Bus: MscpBus_SC4191_5110k_10k
  Bus Selector1 : BusSelector  OutputSignals=Channel_01
  S-Function1 : S-Function  FunctionName=sg_mscp_SC4191_5110k_10k_write  SFunctionDeploymentMode=off  EnableBusSupport=off
  exp0bank0 : slrealtimeethercatlib/EtherCAT PDO Transmit  Priority=3  sig_name=Uninitialized Block  sig_offset=128  sig_type=uint8  type_size=8  sig_dim=1  device_id=0  sample_time=0.010000
  exp0bank1 : slrealtimeethercatlib/EtherCAT PDO Transmit  Priority=3  sig_name=Uninitialized Block  sig_offset=128  sig_type=uint8  type_size=8  sig_dim=1  device_id=0  sample_time=0.010000
  wires:
  Bus Selector1/1 -> S-Function1/1  "<Channel_01>"
  In2/1 -> Bus Selector1/1
  S-Function1/2 -> exp0bank1/1
  S-Function1/1 -> exp0bank0/1

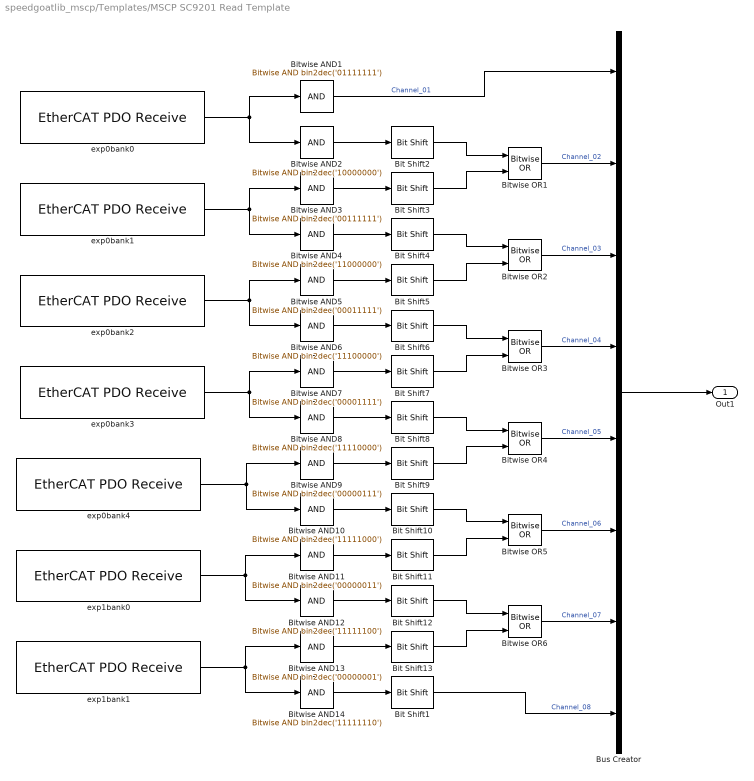
== system speedgoatlib_mscp/Templates/MSCP SC9201 Read Template ==
  Bit Shift1 : hdlsllib/Logic and Bit Operations/Bit Shift  mode=Shift Right Logical  N=1
  Bit Shift10 : hdlsllib/Logic and Bit Operations/Bit Shift  mode=Shift Right Logical  N=3
  Bit Shift11 : hdlsllib/Logic and Bit Operations/Bit Shift  mode=Shift Left Logical  N=5
  Bit Shift12 : hdlsllib/Logic and Bit Operations/Bit Shift  mode=Shift Right Logical  N=2
  Bit Shift13 : hdlsllib/Logic and Bit Operations/Bit Shift  mode=Shift Left Logical  N=6
  Bit Shift2 : hdlsllib/Logic and Bit Operations/Bit Shift  mode=Shift Right Logical  N=7
  Bit Shift3 : hdlsllib/Logic and Bit Operations/Bit Shift  mode=Shift Left Logical  N=1
  Bit Shift4 : hdlsllib/Logic and Bit Operations/Bit Shift  mode=Shift Right Logical  N=6
  Bit Shift5 : hdlsllib/Logic and Bit Operations/Bit Shift  mode=Shift Left Logical  N=2
  Bit Shift6 : hdlsllib/Logic and Bit Operations/Bit Shift  mode=Shift Right Logical  N=5
  Bit Shift7 : hdlsllib/Logic and Bit Operations/Bit Shift  mode=Shift Left Logical  N=3
  Bit Shift8 : hdlsllib/Logic and Bit Operations/Bit Shift  mode=Shift Right Logical  N=4
  Bit Shift9 : hdlsllib/Logic and Bit Operations/Bit Shift  mode=Shift Left Logical  N=4
  Bitwise AND1 : simulink/Logic and Bit Operations/Bitwise Operator  logicop=AND  UseBitMask=on  BitMask=bin2dec('01111111')  BitMaskRealWorld=Stored Integer
      settings: LibrarySourceBlock=|
      | simulink/Quick Insert/Logic and Bit
      | Operations/Bitwise AND
  Bitwise AND10 : simulink/Logic and Bit Operations/Bitwise Operator  logicop=AND  UseBitMask=on  BitMask=bin2dec('11111000')  BitMaskRealWorld=Stored Integer
      settings: LibrarySourceBlock=|
      | simulink/Quick Insert/Logic and Bit
      | Operations/Bitwise AND
  Bitwise AND11 : simulink/Logic and Bit Operations/Bitwise Operator  logicop=AND  UseBitMask=on  BitMask=bin2dec('00000011')  BitMaskRealWorld=Stored Integer
      settings: LibrarySourceBlock=|
      | simulink/Quick Insert/Logic and Bit
      | Operations/Bitwise AND
  Bitwise AND12 : simulink/Logic and Bit Operations/Bitwise Operator  logicop=AND  UseBitMask=on  BitMask=bin2dec('11111100')  BitMaskRealWorld=Stored Integer
      settings: LibrarySourceBlock=|
      | simulink/Quick Insert/Logic and Bit
      | Operations/Bitwise AND
  Bitwise AND13 : simulink/Logic and Bit Operations/Bitwise Operator  logicop=AND  UseBitMask=on  BitMask=bin2dec('00000001')  BitMaskRealWorld=Stored Integer
      settings: LibrarySourceBlock=|
      | simulink/Quick Insert/Logic and Bit
      | Operations/Bitwise AND
  Bitwise AND14 : simulink/Logic and Bit Operations/Bitwise Operator  logicop=AND  UseBitMask=on  BitMask=bin2dec('11111110')  BitMaskRealWorld=Stored Integer
      settings: LibrarySourceBlock=|
      | simulink/Quick Insert/Logic and Bit
      | Operations/Bitwise AND
  Bitwise AND2 : simulink/Logic and Bit Operations/Bitwise Operator  logicop=AND  UseBitMask=on  BitMask=bin2dec('10000000')  BitMaskRealWorld=Stored Integer
      settings: LibrarySourceBlock=|
      | simulink/Quick Insert/Logic and Bit
      | Operations/Bitwise AND
  Bitwise AND3 : simulink/Logic and Bit Operations/Bitwise Operator  logicop=AND  UseBitMask=on  BitMask=bin2dec('00111111')  BitMaskRealWorld=Stored Integer
      settings: LibrarySourceBlock=|
      | simulink/Quick Insert/Logic and Bit
      | Operations/Bitwise AND
  Bitwise AND4 : simulink/Logic and Bit Operations/Bitwise Operator  logicop=AND  UseBitMask=on  BitMask=bin2dec('11000000')  BitMaskRealWorld=Stored Integer
      settings: LibrarySourceBlock=|
      | simulink/Quick Insert/Logic and Bit
      | Operations/Bitwise AND
  Bitwise AND5 : simulink/Logic and Bit Operations/Bitwise Operator  logicop=AND  UseBitMask=on  BitMask=bin2dec('00011111')  BitMaskRealWorld=Stored Integer
      settings: LibrarySourceBlock=|
      | simulink/Quick Insert/Logic and Bit
      | Operations/Bitwise AND
  Bitwise AND6 : simulink/Logic and Bit Operations/Bitwise Operator  logicop=AND  UseBitMask=on  BitMask=bin2dec('11100000')  BitMaskRealWorld=Stored Integer
      settings: LibrarySourceBlock=|
      | simulink/Quick Insert/Logic and Bit
      | Operations/Bitwise AND
  Bitwise AND7 : simulink/Logic and Bit Operations/Bitwise Operator  logicop=AND  UseBitMask=on  BitMask=bin2dec('00001111')  BitMaskRealWorld=Stored Integer
      settings: LibrarySourceBlock=|
      | simulink/Quick Insert/Logic and Bit
      | Operations/Bitwise AND
  Bitwise AND8 : simulink/Logic and Bit Operations/Bitwise Operator  logicop=AND  UseBitMask=on  BitMask=bin2dec('11110000')  BitMaskRealWorld=Stored Integer
      settings: LibrarySourceBlock=|
      | simulink/Quick Insert/Logic and Bit
      | Operations/Bitwise AND
  Bitwise AND9 : simulink/Logic and Bit Operations/Bitwise Operator  logicop=AND  UseBitMask=on  BitMask=bin2dec('00000111')  BitMaskRealWorld=Stored Integer
      settings: LibrarySourceBlock=|
      | simulink/Quick Insert/Logic and Bit
      | Operations/Bitwise AND
  Bitwise OR{1..6} (6 alike) : simulink/Logic and Bit Operations/Bitwise Operator  logicop=OR  UseBitMask=off  NumInputPorts=2  BitMask=bin2dec('11011001')  BitMaskRealWorld=Stored Integer
      settings: LibrarySourceBlock=|
      | simulink/Quick Insert/Logic and Bit
      | Operations/Bitwise OR
  Bus Creator : BusCreator  Inputs=8  OutDataTypeStr=Bus: MscpBus_SC9201
      settings: InheritFromInputs=off
  exp0bank{0..4} (5 alike) : slrealtimeethercatlib/EtherCAT PDO Receive  Priority=2  sig_name=Uninitialized Block  sig_offset=144  sig_type=uint8  type_size=8  sig_dim=1  device_id=0  sample_time=0.010000
  exp1bank0 : slrealtimeethercatlib/EtherCAT PDO Receive  Priority=2  sig_name=Uninitialized Block  sig_offset=144  sig_type=uint8  type_size=8  sig_dim=1  device_id=0  sample_time=0.010000
  exp1bank1 : slrealtimeethercatlib/EtherCAT PDO Receive  Priority=2  sig_name=Uninitialized Block  sig_offset=144  sig_type=uint8  type_size=8  sig_dim=1  device_id=0  sample_time=0.010000
  Out1 : Outport
  wires:
  Bus Creator/1 -> Out1/1
  Bitwise AND3/1 -> Bit Shift3/1
  Bitwise OR5/1 -> Bus Creator/6  "Channel_06"
  Bitwise OR2/1 -> Bus Creator/3  "Channel_03"
  Bitwise AND9/1 -> Bit Shift9/1
  Bitwise AND4/1 -> Bit Shift4/1
  Bitwise OR4/1 -> Bus Creator/5  "Channel_05"
  Bitwise AND5/1 -> Bit Shift5/1
  Bitwise AND2/1 -> Bit Shift2/1
  Bitwise AND12/1 -> Bit Shift12/1
  Bit Shift12/1 -> Bitwise OR6/1
  Bitwise AND1/1 -> Bus Creator/1  "Channel_01"
  Bit Shift6/1 -> Bitwise OR3/1
  Bitwise AND11/1 -> Bit Shift11/1
  Bitwise AND10/1 -> Bit Shift10/1
  Bit Shift4/1 -> Bitwise OR2/1
  Bit Shift5/1 -> Bitwise OR2/2
  Bitwise AND7/1 -> Bit Shift7/1
  Bitwise OR3/1 -> Bus Creator/4  "Channel_04"
  Bit Shift8/1 -> Bitwise OR4/1
  Bit Shift11/1 -> Bitwise OR5/2
  Bitwise AND13/1 -> Bit Shift13/1
  Bit Shift13/1 -> Bitwise OR6/2
  Bit Shift10/1 -> Bitwise OR5/1
  Bitwise OR1/1 -> Bus Creator/2  "Channel_02"
  Bitwise AND6/1 -> Bit Shift6/1
  Bitwise AND8/1 -> Bit Shift8/1
  Bit Shift7/1 -> Bitwise OR3/2
  Bit Shift3/1 -> Bitwise OR1/2
  Bit Shift2/1 -> Bitwise OR1/1
  Bitwise OR6/1 -> Bus Creator/7  "Channel_07"
  Bit Shift9/1 -> Bitwise OR4/2
  exp0bank0/1 -> Bitwise AND2/1, Bitwise AND1/1
  exp0bank1/1 -> Bitwise AND3/1, Bitwise AND4/1
  exp0bank2/1 -> Bitwise AND5/1, Bitwise AND6/1
  exp0bank3/1 -> Bitwise AND8/1, Bitwise AND7/1
  exp0bank4/1 -> Bitwise AND10/1, Bitwise AND9/1
  exp1bank0/1 -> Bitwise AND11/1, Bitwise AND12/1
  exp1bank1/1 -> Bitwise AND14/1, Bitwise AND13/1
  Bitwise AND14/1 -> Bit Shift1/1
  Bit Shift1/1 -> Bus Creator/8  "Channel_08"

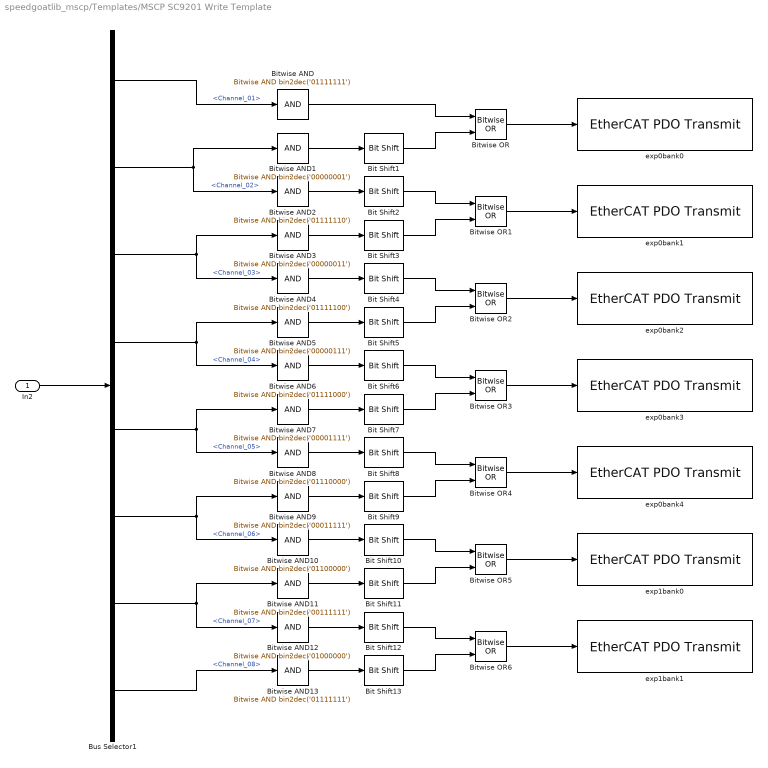
== system speedgoatlib_mscp/Templates/MSCP SC9201 Write Template ==
  In2 : Inport  OutDataTypeStr=Bus: MscpBus_SC9201
  Bit Shift1 : hdlsllib/Logic and Bit Operations/Bit Shift  mode=Shift Left Logical  N=7
  Bit Shift10 : hdlsllib/Logic and Bit Operations/Bit Shift  mode=Shift Right Logical  N=5
  Bit Shift11 : hdlsllib/Logic and Bit Operations/Bit Shift  mode=Shift Left Logical  N=2
  Bit Shift12 : hdlsllib/Logic and Bit Operations/Bit Shift  mode=Shift Right Logical  N=6
  Bit Shift13 : hdlsllib/Logic and Bit Operations/Bit Shift  mode=Shift Left Logical  N=1
  Bit Shift2 : hdlsllib/Logic and Bit Operations/Bit Shift  mode=Shift Right Logical  N=1
  Bit Shift3 : hdlsllib/Logic and Bit Operations/Bit Shift  mode=Shift Left Logical  N=6
  Bit Shift4 : hdlsllib/Logic and Bit Operations/Bit Shift  mode=Shift Right Logical  N=2
  Bit Shift5 : hdlsllib/Logic and Bit Operations/Bit Shift  mode=Shift Left Logical  N=5
  Bit Shift6 : hdlsllib/Logic and Bit Operations/Bit Shift  mode=Shift Right Logical  N=3
  Bit Shift7 : hdlsllib/Logic and Bit Operations/Bit Shift  mode=Shift Left Logical  N=4
  Bit Shift8 : hdlsllib/Logic and Bit Operations/Bit Shift  mode=Shift Right Logical  N=4
  Bit Shift9 : hdlsllib/Logic and Bit Operations/Bit Shift  mode=Shift Left Logical  N=3
  Bitwise AND : simulink/Logic and Bit Operations/Bitwise Operator  logicop=AND  UseBitMask=on  BitMask=bin2dec('01111111')  BitMaskRealWorld=Stored Integer
      settings: LibrarySourceBlock=|
      | simulink/Quick Insert/Logic and Bit
      | Operations/Bitwise AND
  Bitwise AND1 : simulink/Logic and Bit Operations/Bitwise Operator  logicop=AND  UseBitMask=on  BitMask=bin2dec('00000001')  BitMaskRealWorld=Stored Integer
      settings: LibrarySourceBlock=|
      | simulink/Quick Insert/Logic and Bit
      | Operations/Bitwise AND
  Bitwise AND10 : simulink/Logic and Bit Operations/Bitwise Operator  logicop=AND  UseBitMask=on  BitMask=bin2dec('01100000')  BitMaskRealWorld=Stored Integer
      settings: LibrarySourceBlock=|
      | simulink/Quick Insert/Logic and Bit
      | Operations/Bitwise AND
  Bitwise AND11 : simulink/Logic and Bit Operations/Bitwise Operator  logicop=AND  UseBitMask=on  BitMask=bin2dec('00111111')  BitMaskRealWorld=Stored Integer
      settings: LibrarySourceBlock=|
      | simulink/Quick Insert/Logic and Bit
      | Operations/Bitwise AND
  Bitwise AND12 : simulink/Logic and Bit Operations/Bitwise Operator  logicop=AND  UseBitMask=on  BitMask=bin2dec('01000000')  BitMaskRealWorld=Stored Integer
      settings: LibrarySourceBlock=|
      | simulink/Quick Insert/Logic and Bit
      | Operations/Bitwise AND
  Bitwise AND13 : simulink/Logic and Bit Operations/Bitwise Operator  logicop=AND  UseBitMask=on  BitMask=bin2dec('01111111')  BitMaskRealWorld=Stored Integer
      settings: LibrarySourceBlock=|
      | simulink/Quick Insert/Logic and Bit
      | Operations/Bitwise AND
  Bitwise AND2 : simulink/Logic and Bit Operations/Bitwise Operator  logicop=AND  UseBitMask=on  BitMask=bin2dec('01111110')  BitMaskRealWorld=Stored Integer
      settings: LibrarySourceBlock=|
      | simulink/Quick Insert/Logic and Bit
      | Operations/Bitwise AND
  Bitwise AND3 : simulink/Logic and Bit Operations/Bitwise Operator  logicop=AND  UseBitMask=on  BitMask=bin2dec('00000011')  BitMaskRealWorld=Stored Integer
      settings: LibrarySourceBlock=|
      | simulink/Quick Insert/Logic and Bit
      | Operations/Bitwise AND
  Bitwise AND4 : simulink/Logic and Bit Operations/Bitwise Operator  logicop=AND  UseBitMask=on  BitMask=bin2dec('01111100')  BitMaskRealWorld=Stored Integer
      settings: LibrarySourceBlock=|
      | simulink/Quick Insert/Logic and Bit
      | Operations/Bitwise AND
  Bitwise AND5 : simulink/Logic and Bit Operations/Bitwise Operator  logicop=AND  UseBitMask=on  BitMask=bin2dec('00000111')  BitMaskRealWorld=Stored Integer
      settings: LibrarySourceBlock=|
      | simulink/Quick Insert/Logic and Bit
      | Operations/Bitwise AND
  Bitwise AND6 : simulink/Logic and Bit Operations/Bitwise Operator  logicop=AND  UseBitMask=on  BitMask=bin2dec('01111000')  BitMaskRealWorld=Stored Integer
      settings: LibrarySourceBlock=|
      | simulink/Quick Insert/Logic and Bit
      | Operations/Bitwise AND
  Bitwise AND7 : simulink/Logic and Bit Operations/Bitwise Operator  logicop=AND  UseBitMask=on  BitMask=bin2dec('00001111')  BitMaskRealWorld=Stored Integer
      settings: LibrarySourceBlock=|
      | simulink/Quick Insert/Logic and Bit
      | Operations/Bitwise AND
  Bitwise AND8 : simulink/Logic and Bit Operations/Bitwise Operator  logicop=AND  UseBitMask=on  BitMask=bin2dec('01110000')  BitMaskRealWorld=Stored Integer
      settings: LibrarySourceBlock=|
      | simulink/Quick Insert/Logic and Bit
      | Operations/Bitwise AND
  Bitwise AND9 : simulink/Logic and Bit Operations/Bitwise Operator  logicop=AND  UseBitMask=on  BitMask=bin2dec('00011111')  BitMaskRealWorld=Stored Integer
      settings: LibrarySourceBlock=|
      | simulink/Quick Insert/Logic and Bit
      | Operations/Bitwise AND
  Bitwise OR{,1..6} (7 alike) : simulink/Logic and Bit Operations/Bitwise Operator  logicop=OR  UseBitMask=off  NumInputPorts=2  BitMask=bin2dec('11011001')  BitMaskRealWorld=Stored Integer
      settings: LibrarySourceBlock=|
      | simulink/Quick Insert/Logic and Bit
      | Operations/Bitwise OR
  Bus Selector1 : BusSelector  OutputSignals=Channel_01,Channel_02,Channel_03,Channel_04,Channel_05,Channel_06,Channel_07,Channel_08
  exp0bank{0..4} (5 alike) : slrealtimeethercatlib/EtherCAT PDO Transmit  Priority=3  sig_name=Uninitialized Block  sig_offset=128  sig_type=uint8  type_size=8  sig_dim=1  device_id=0  sample_time=0.010000
  exp1bank0 : slrealtimeethercatlib/EtherCAT PDO Transmit  Priority=3  sig_name=Uninitialized Block  sig_offset=128  sig_type=uint8  type_size=8  sig_dim=1  device_id=0  sample_time=0.010000
  exp1bank1 : slrealtimeethercatlib/EtherCAT PDO Transmit  Priority=3  sig_name=Uninitialized Block  sig_offset=128  sig_type=uint8  type_size=8  sig_dim=1  device_id=0  sample_time=0.010000
  wires:
  Bitwise OR1/1 -> exp0bank1/1
  Bitwise AND8/1 -> Bit Shift8/1
  Bit Shift13/1 -> Bitwise OR6/2
  Bit Shift7/1 -> Bitwise OR3/2
  Bit Shift10/1 -> Bitwise OR5/1
  Bit Shift8/1 -> Bitwise OR4/1
  Bus Selector1/8 -> Bitwise AND13/1  "<Channel_08>"
  Bit Shift4/1 -> Bitwise OR2/1
  Bitwise AND7/1 -> Bit Shift7/1
  Bus Selector1/7 -> Bitwise AND12/1, Bitwise AND11/1  "<Channel_07>"
  Bit Shift6/1 -> Bitwise OR3/1
  Bitwise AND11/1 -> Bit Shift11/1
  Bitwise OR6/1 -> exp1bank1/1
  Bit Shift3/1 -> Bitwise OR1/2
  Bitwise AND/1 -> Bitwise OR/1
  Bitwise AND12/1 -> Bit Shift12/1
  Bitwise AND10/1 -> Bit Shift10/1
  Bitwise AND2/1 -> Bit Shift2/1
  Bit Shift1/1 -> Bitwise OR/2
  Bit Shift11/1 -> Bitwise OR5/2
  Bus Selector1/6 -> Bitwise AND10/1, Bitwise AND9/1  "<Channel_06>"
  Bitwise OR3/1 -> exp0bank3/1
  Bus Selector1/4 -> Bitwise AND6/1, Bitwise AND5/1  "<Channel_04>"
  Bus Selector1/3 -> Bitwise AND4/1, Bitwise AND3/1  "<Channel_03>"
  Bus Selector1/1 -> Bitwise AND/1  "<Channel_01>"
  Bitwise AND1/1 -> Bit Shift1/1
  Bit Shift2/1 -> Bitwise OR1/1
  Bitwise OR4/1 -> exp0bank4/1
  Bitwise AND5/1 -> Bit Shift5/1
  In2/1 -> Bus Selector1/1
  Bitwise AND9/1 -> Bit Shift9/1
  Bitwise AND4/1 -> Bit Shift4/1
  Bit Shift12/1 -> Bitwise OR6/1
  Bitwise AND13/1 -> Bit Shift13/1
  Bus Selector1/5 -> Bitwise AND8/1, Bitwise AND7/1  "<Channel_05>"
  Bit Shift5/1 -> Bitwise OR2/2
  Bit Shift9/1 -> Bitwise OR4/2
  Bitwise OR/1 -> exp0bank0/1
  Bitwise OR2/1 -> exp0bank2/1
  Bitwise AND3/1 -> Bit Shift3/1
  Bitwise AND6/1 -> Bit Shift6/1
  Bitwise OR5/1 -> exp1bank0/1
  Bus Selector1/2 -> Bitwise AND2/1, Bitwise AND1/1  "<Channel_02>"
